simulink model "IEEE30_case"  (R2024b)
settings: Solver=FixedStepAuto  StartTime=0  StopTime=5  FixedStep=1e-7  RelTol=1e-3
values from neighbouring files (symbols this model uses):
  GFL_DFIG_7_C_bus = 0.08    [IEEE30_case_parameters.m]
  GFL_DFIG_7_D_mutual = 2.500000e+3    (= 2500)    [IEEE30_case_parameters.m]
  GFL_DFIG_7_f0 = 60    [IEEE30_case_parameters.m]
  GFL_DFIG_7_gPLLi = 3200    [IEEE30_case_parameters.m]
  GFL_DFIG_7_gPLLp = 650    [IEEE30_case_parameters.m]
  GFL_DFIG_7_H_WT = 0.4    [IEEE30_case_parameters.m]
  GFL_DFIG_7_Hg = 0.8    [IEEE30_case_parameters.m]
  GFL_DFIG_7_Igq_ref = 0    [IEEE30_case_parameters.m]
  GFL_DFIG_7_Ird_ref = 704.45696    [IEEE30_case_parameters.m]
  GFL_DFIG_7_KI_V = -300000    [IEEE30_case_parameters.m]
  GFL_DFIG_7_KP_V = -1000    [IEEE30_case_parameters.m]
  GFL_DFIG_7_Ksh = 1.254300e+4    (= 12543)    [IEEE30_case_parameters.m]
  GFL_DFIG_7_Lg = 0.000483    [IEEE30_case_parameters.m]
  GFL_DFIG_7_Lm_pu = 4    [IEEE30_case_parameters.m]
  GFL_DFIG_7_N = 100    [IEEE30_case_parameters.m]
  GFL_DFIG_7_p = 2    [IEEE30_case_parameters.m]
  GFL_DFIG_7_Pitch = 0    [IEEE30_case_parameters.m]
  GFL_DFIG_7_R = 44    [IEEE30_case_parameters.m]
  GFL_DFIG_7_Rg = 2.000000e-5    (= 2e-05)    [IEEE30_case_parameters.m]
  GFL_DFIG_7_rho = 1.225    [IEEE30_case_parameters.m]
  GFL_DFIG_7_rPLLi = 4500    [IEEE30_case_parameters.m]
  GFL_DFIG_7_rPLLp = 620    [IEEE30_case_parameters.m]
  GFL_DFIG_7_Rs_pu = 0.011    [IEEE30_case_parameters.m]
  GFL_DFIG_7_Sbase = 2.000000e+6    (= 2000000)    [IEEE30_case_parameters.m]
  GFL_DFIG_7_ugq_ref = 0    [IEEE30_case_parameters.m]
  GFL_DFIG_7_usd_ref = 0    [IEEE30_case_parameters.m]
  GFL_DFIG_7_Vbase = 690    [IEEE30_case_parameters.m]
  GFL_DFIG_7_Vdc_ref = 1200    [IEEE30_case_parameters.m]
  GFL_DFIG_7_wind = 12    [IEEE30_case_parameters.m]
  GFL_DFIG_7_wm_ref = 518.184209    [IEEE30_case_parameters.m]
  SG_D_13_D = 0.01056    [IEEE30_case_parameters.m]
  SG_D_13_EnableSaturation = 0    [IEEE30_case_parameters.m]
  SG_D_13_f0 = 60    [IEEE30_case_parameters.m]
  SG_D_13_H = 7.5    [IEEE30_case_parameters.m]
  SG_D_13_K_A = 20    [IEEE30_case_parameters.m]
  SG_D_13_K_E = 1.000000e+1    (= 10)    [IEEE30_case_parameters.m]
  SG_D_13_K_F = 2.363    [IEEE30_case_parameters.m]
  SG_D_13_K_s = 0.5    [IEEE30_case_parameters.m]
  SG_D_13_R_a = 0.001088    [IEEE30_case_parameters.m]
  SG_D_13_S_A = 1    [IEEE30_case_parameters.m]
  SG_D_13_S_B = 0.103    [IEEE30_case_parameters.m]
  SG_D_13_S_N = 10.659857    [IEEE30_case_parameters.m]
  SG_D_13_SpeedPara = 200    [IEEE30_case_parameters.m]
  SG_D_13_T_0 = 0.370163    [IEEE30_case_parameters.m]
  SG_D_13_T_1 = 0.3    [IEEE30_case_parameters.m]
  SG_D_13_T_2 = 0.05    [IEEE30_case_parameters.m]
  SG_D_13_T_3 = 0.02    [IEEE30_case_parameters.m]
  SG_D_13_T_4 = 0.005    [IEEE30_case_parameters.m]
  SG_D_13_T_A = 0.02    [IEEE30_case_parameters.m]
  SG_D_13_T_dd = 8.000000e+0    (= 8)    [IEEE30_case_parameters.m]
  SG_D_13_T_ddd = 0.04    [IEEE30_case_parameters.m]
  SG_D_13_T_E = 0.314    [IEEE30_case_parameters.m]
  SG_D_13_T_F = 0.35    [IEEE30_case_parameters.m]
  SG_D_13_T_qd = 0.8    [IEEE30_case_parameters.m]
  SG_D_13_T_qdd = 0.02    [IEEE30_case_parameters.m]
  SG_D_13_T_speed = 0.1    [IEEE30_case_parameters.m]
  SG_D_13_T_w = 0.5    [IEEE30_case_parameters.m]
  SG_D_13_V_ref = 1.696619    [IEEE30_case_parameters.m]
  SG_D_13_w_ref = 376.991118    [IEEE30_case_parameters.m]
  SG_D_13_x_d = 1.9    [IEEE30_case_parameters.m]
  SG_D_13_x_dd = 0.302    [IEEE30_case_parameters.m]
  SG_D_13_x_ddd = 0.204    [IEEE30_case_parameters.m]
  SG_D_13_x_l = 0.05    [IEEE30_case_parameters.m]
  SG_D_13_x_q = 1.3    [IEEE30_case_parameters.m]
  SG_D_13_x_qd = 0.5    [IEEE30_case_parameters.m]
  SG_D_13_x_qdd = 0.3    [IEEE30_case_parameters.m]
  SG_D_1_D = 0.01056    [IEEE30_case_parameters.m]
  SG_D_1_EnableSaturation = 0    [IEEE30_case_parameters.m]
  SG_D_1_f0 = 60    [IEEE30_case_parameters.m]
  SG_D_1_H = 7.5    [IEEE30_case_parameters.m]
  SG_D_1_K_A = 20    [IEEE30_case_parameters.m]
  SG_D_1_K_E = 1.000000e+1    (= 10)    [IEEE30_case_parameters.m]
  SG_D_1_K_F = 2.363    [IEEE30_case_parameters.m]
  SG_D_1_K_s = 0.5    [IEEE30_case_parameters.m]
  SG_D_1_R_a = 0.001088    [IEEE30_case_parameters.m]
  SG_D_1_S_A = 1    [IEEE30_case_parameters.m]
  SG_D_1_S_B = 0.103    [IEEE30_case_parameters.m]
  SG_D_1_S_N = 10.659857    [IEEE30_case_parameters.m]
  SG_D_1_SpeedPara = 200    [IEEE30_case_parameters.m]
  SG_D_1_T_0 = 0.259812    [IEEE30_case_parameters.m]
  SG_D_1_T_1 = 0.3    [IEEE30_case_parameters.m]
  SG_D_1_T_2 = 0.05    [IEEE30_case_parameters.m]
  SG_D_1_T_3 = 0.02    [IEEE30_case_parameters.m]
  SG_D_1_T_4 = 0.005    [IEEE30_case_parameters.m]
  SG_D_1_T_A = 0.02    [IEEE30_case_parameters.m]
  SG_D_1_T_dd = 8.000000e+0    (= 8)    [IEEE30_case_parameters.m]
  SG_D_1_T_ddd = 0.04    [IEEE30_case_parameters.m]
  SG_D_1_T_E = 0.314    [IEEE30_case_parameters.m]
  SG_D_1_T_F = 0.35    [IEEE30_case_parameters.m]
  SG_D_1_T_qd = 0.8    [IEEE30_case_parameters.m]
  SG_D_1_T_qdd = 0.02    [IEEE30_case_parameters.m]
  SG_D_1_T_speed = 0.1    [IEEE30_case_parameters.m]
  SG_D_1_T_w = 0.5    [IEEE30_case_parameters.m]
  SG_D_1_V_ref = 1.544107    [IEEE30_case_parameters.m]
  SG_D_1_w_ref = 376.991118    [IEEE30_case_parameters.m]
  SG_D_1_x_d = 1.9    [IEEE30_case_parameters.m]
  SG_D_1_x_dd = 0.302    [IEEE30_case_parameters.m]
  SG_D_1_x_ddd = 0.204    [IEEE30_case_parameters.m]
  SG_D_1_x_l = 0.05    [IEEE30_case_parameters.m]
  SG_D_1_x_q = 1.3    [IEEE30_case_parameters.m]
  SG_D_1_x_qd = 0.5    [IEEE30_case_parameters.m]
  SG_D_1_x_qdd = 0.3    [IEEE30_case_parameters.m]
  SG_D_22_D = 0.01056    [IEEE30_case_parameters.m]
  SG_D_22_EnableSaturation = 0    [IEEE30_case_parameters.m]
  SG_D_22_f0 = 60    [IEEE30_case_parameters.m]
  SG_D_22_H = 7.5    [IEEE30_case_parameters.m]
  SG_D_22_K_A = 20    [IEEE30_case_parameters.m]
  SG_D_22_K_E = 1.000000e+1    (= 10)    [IEEE30_case_parameters.m]
  SG_D_22_K_F = 2.363    [IEEE30_case_parameters.m]
  SG_D_22_K_s = 0.5    [IEEE30_case_parameters.m]
  SG_D_22_R_a = 0.001088    [IEEE30_case_parameters.m]
  SG_D_22_S_A = 1    [IEEE30_case_parameters.m]
  SG_D_22_S_B = 0.103    [IEEE30_case_parameters.m]
  SG_D_22_S_N = 10.659857    [IEEE30_case_parameters.m]
  SG_D_22_SpeedPara = 200    [IEEE30_case_parameters.m]
  SG_D_22_T_0 = 0.216121    [IEEE30_case_parameters.m]
  SG_D_22_T_1 = 0.3    [IEEE30_case_parameters.m]
  SG_D_22_T_2 = 0.05    [IEEE30_case_parameters.m]
  SG_D_22_T_3 = 0.02    [IEEE30_case_parameters.m]
  SG_D_22_T_4 = 0.005    [IEEE30_case_parameters.m]
  ... (+126 more)
(part 17 of 27)

== system IEEE30_case/SG_D_1/d_psi_kq_SG_D_1_block ==
  note: d_psi_kq_SG_D_1 in IEEE30_case
      | $-\frac{\psi _{\mathrm{gq},\mathrm{SG},D,1}+\psi _{\mathrm{kq},\mathrm{SG},D,1}+\frac{\left(x_{l}-x_{\mathrm{qd}}\right)\,\left(\psi _{q,\mathrm{SG},D,1}+\frac{\psi _{\mathrm{gq},\mathrm{SG},D,1}\,\left(x_{l}-x_{\mathrm{qdd}}\right)}{x_{l}-x_{\mathrm{qd}}}+\frac{\psi _{\mathrm{kq},\mathrm{SG},D,1}\,\left(x_{\mathrm{qd}}-x_{\mathrm{qdd}}\right)}{x_{l}-x_{\mathrm{qd}}}\right)}{x_{\mathrm{qdd}}}}{T_{\mathrm{qdd}}}$
      | Automatically generated on 2025-11-01 18:30:18 .
  State_psi_gq_SG_D_1_66a42 : Inport
  State_psi_kq_SG_D_1_f6edb : Inport  Port=2
  State_psi_gq_SG_D_1_3bf06 : Inport  Port=3
  State_psi_kq_SG_D_1_b2a24 : Inport  Port=4
  State_psi_q_SG_D_1_f72b4 : Inport  Port=5
  Add_37b64 : Sum
  Add_70e19 : Sum
  Add_86bb6 : Sum
  Add_caec9 : Sum
  Add_e8957 : Sum
  Add_f96b5 : Sum
  Constant_-1_1ee71 : Constant  Value=-1
  Constant_-1_42dcf : Constant  Value=-1
  Constant_-1_ae184 : Constant  Value=-1
  Constant_-1_b39c3 : Constant  Value=-1
  Constant_-1_df8ac : Constant  Value=-1
  Constant_T_qdd_72f05 : Constant  Value=T_qdd
  Constant_x_l_0c777 : Constant  Value=x_l
  Constant_x_l_15b0a : Constant  Value=x_l
  Constant_x_l_3ca11 : Constant  Value=x_l
  Constant_x_l_4ff6a : Constant  Value=x_l
  Constant_x_qd_677f8 : Constant  Value=x_qd
  Constant_x_qd_b6ebb : Constant  Value=x_qd
  Constant_x_qd_d4607 : Constant  Value=x_qd
  Constant_x_qd_dcc1d : Constant  Value=x_qd
  Constant_x_qdd_61ea3 : Constant  Value=x_qdd
  Constant_x_qdd_8287c : Constant  Value=x_qdd
  Constant_x_qdd_95e13 : Constant  Value=x_qdd
  Divide_1c15d : Product  Inputs=*/
  Divide_39d85 : Product  Inputs=*/
  Divide_cbd1b : Product  Inputs=*/
  Divide_e3ee2 : Product  Inputs=*/
  Product_05f1c : Product
  Product_6315e : Product
  Product_6a7e9 : Product
  Product_6f561 : Product
  Product_70210 : Product
  Product_d8668 : Product
  Product_e096e : Product
  Product_f70fb : Product
  Subtract_2999a : Sum  Inputs=+-
  Subtract_5330c : Sum  Inputs=+-
  Subtract_efeff : Sum  Inputs=+-
  Blockout_d_psi_kq_SG_D_1_05b7c : Outport
  wires:
  Product_6f561/1 -> Add_caec9/1
  Constant_-1_ae184/1 -> Product_6f561/1
  Constant_x_l_15b0a/1 -> Product_6f561/2
  Constant_x_qdd_95e13/1 -> Add_caec9/2
  Constant_-1_df8ac/1 -> Product_70210/1
  Constant_x_qd_677f8/1 -> Subtract_5330c/1
  Constant_x_qd_d4607/1 -> Add_86bb6/2
  Constant_-1_1ee71/1 -> Product_e096e/1
  Constant_x_l_4ff6a/1 -> Product_70210/2
  Constant_x_qdd_8287c/1 -> Subtract_5330c/2
  Constant_x_qd_b6ebb/1 -> Add_f96b5/2
  Constant_x_l_0c777/1 -> Product_e096e/2
  Subtract_2999a/1 -> Add_37b64/1
  Product_f70fb/1 -> Subtract_2999a/1
  State_psi_gq_SG_D_1_3bf06/1 -> Product_d8668/1
  Add_caec9/1 -> Product_d8668/2
  Product_e096e/1 -> Add_e8957/1
  Constant_x_qd_dcc1d/1 -> Add_e8957/2
  State_psi_kq_SG_D_1_b2a24/1 -> Product_05f1c/1
  Product_70210/1 -> Add_f96b5/1
  Subtract_5330c/1 -> Product_05f1c/2
  Product_d8668/1 -> Divide_e3ee2/1
  Add_e8957/1 -> Divide_e3ee2/2
  Product_05f1c/1 -> Divide_39d85/1
  Add_f96b5/1 -> Divide_39d85/2
  Constant_-1_b39c3/1 -> Product_6315e/1
  Constant_x_l_3ca11/1 -> Product_6315e/2
  Divide_e3ee2/1 -> Subtract_efeff/1
  Divide_39d85/1 -> Subtract_efeff/2
  Product_6315e/1 -> Add_86bb6/1
  Add_70e19/1 -> Product_6a7e9/2
  Subtract_efeff/1 -> Add_70e19/1
  State_psi_q_SG_D_1_f72b4/1 -> Add_70e19/2
  Constant_-1_42dcf/1 -> Product_f70fb/1
  State_psi_gq_SG_D_1_66a42/1 -> Product_f70fb/2
  Divide_1c15d/1 -> Add_37b64/2
  Product_6a7e9/1 -> Divide_1c15d/1
  Add_86bb6/1 -> Product_6a7e9/1
  State_psi_kq_SG_D_1_f6edb/1 -> Subtract_2999a/2
  Constant_x_qdd_61ea3/1 -> Divide_1c15d/2
  Add_37b64/1 -> Divide_cbd1b/1
  Constant_T_qdd_72f05/1 -> Divide_cbd1b/2
  Divide_cbd1b/1 -> Blockout_d_psi_kq_SG_D_1_05b7c/1

== system IEEE30_case/SG_D_1/d_psi_q_SG_D_1_block ==
  note: d_psi_q_SG_D_1 in IEEE30_case
      | $2\,\pi \,f_{0}\,\left(v_{d,\mathrm{SG},D,1}\,\cos\left(\theta _{\mathrm{SG},D,1}\right)+v_{q,\mathrm{SG},D,1}\,\sin\left(\theta _{\mathrm{SG},D,1}\right)-\frac{R_{a}\,\left(\psi _{q,\mathrm{SG},D,1}+\frac{\psi _{\mathrm{gq},\mathrm{SG},D,1}\,\left(x_{l}-x_{\mathrm{qdd}}\right)}{x_{l}-x_{\mathrm{qd}}}+\frac{\psi _{\mathrm{kq},\mathrm{SG},D,1}\,\left(x_{\mathrm{qd}}-x_{\mathrm{qdd}}\right)}{x_{l}-x_{\mathrm{qd}}}\right)}{x_{\mathrm{qdd}}}-\frac{\psi _{d,\mathrm{SG},D,1}\,w_{\mathrm{SG},D,1}}{2\,f_{0}\,\pi }\right)$
      | Automatically generated on 2025-11-01 18:30:00 .
  State_psi_gq_SG_D_1_26e24 : Inport
  State_psi_kq_SG_D_1_f77dd : Inport  Port=2
  State_psi_q_SG_D_1_070ab : Inport  Port=3
  Input_v_d_SG_D_1_1c698 : Inport  Port=4
  State_theta_SG_D_1_9525e : Inport  Port=5
  Input_v_q_SG_D_1_e75ba : Inport  Port=6
  State_theta_SG_D_1_5ff34 : Inport  Port=7
  State_psi_d_SG_D_1_80a58 : Inport  Port=8
  State_w_SG_D_1_948ae : Inport  Port=9
  Add_13797 : Sum
  Add_7e781 : Sum
  Add_babbf : Sum
  Add_e7483 : Sum
  Add_fa18c : Sum
  Constant_-1_3c07d : Constant  Value=-1
  Constant_-1_59b7b : Constant  Value=-1
  Constant_-1_b49b8 : Constant  Value=-1
  Constant_-2.0_d7f57 : Constant  Value=-2.0
  Constant_2.0_efb3f : Constant  Value=2.0
  Constant_R_a_8a746 : Constant  Value=R_a
  Constant_f0_40920 : Constant  Value=f0
  Constant_f0_9936c : Constant  Value=f0
  Constant_pi_9d2f0 : Constant  Value=pi
  Constant_pi_b54fb : Constant  Value=pi
  Constant_x_l_786db : Constant  Value=x_l
  Constant_x_l_8a064 : Constant  Value=x_l
  Constant_x_l_f0cc6 : Constant  Value=x_l
  Constant_x_qd_30d34 : Constant  Value=x_qd
  Constant_x_qd_33bbe : Constant  Value=x_qd
  Constant_x_qd_7c0de : Constant  Value=x_qd
  Constant_x_qdd_2670b : Constant  Value=x_qdd
  Constant_x_qdd_2fe7a : Constant  Value=x_qdd
  Constant_x_qdd_833e6 : Constant  Value=x_qdd
  Divide_25523 : Product  Inputs=*/
  Divide_748df : Product  Inputs=*/
  Divide_82d73 : Product  Inputs=*/
  Divide_b6ace : Product  Inputs=*/
  MathFunc_cos_34627 : Trigonometry  Operator=cos
  MathFunc_sin_db86f : Trigonometry
  Product_09f90 : Product
  Product_7c18a : Product
  Product_813ef : Product
  Product_93581 : Product
  Product_a2672 : Product
  Product_a434f : Product
  Product_c21a3 : Product
  Product_c33c2 : Product
  Product_c7474 : Product
  Product_edeb5 : Product
  Product_f09fe : Product
  Product_f2590 : Product
  Product_f523a : Product
  Product_fbfd0 : Product
  Subtract_2dac9 : Sum  Inputs=+-
  Subtract_4a509 : Sum  Inputs=+-
  Subtract_587b4 : Sum  Inputs=+-
  Subtract_81de1 : Sum  Inputs=+-
  Blockout_d_psi_q_SG_D_1_abfd1 : Outport
  wires:
  Divide_b6ace/1 -> Subtract_587b4/1
  Product_f09fe/1 -> Add_e7483/1
  Constant_x_l_786db/1 -> Product_f09fe/2
  Constant_-1_3c07d/1 -> Product_f09fe/1
  Constant_x_qdd_2fe7a/1 -> Add_e7483/2
  Constant_x_l_f0cc6/1 -> Product_09f90/2
  Constant_-1_b49b8/1 -> Product_09f90/1
  Constant_x_l_8a064/1 -> Product_edeb5/2
  Constant_x_qdd_2670b/1 -> Subtract_81de1/2
  State_psi_kq_SG_D_1_f77dd/1 -> Product_f2590/1
  Constant_-1_59b7b/1 -> Product_edeb5/1
  Constant_x_qd_33bbe/1 -> Subtract_81de1/1
  State_psi_gq_SG_D_1_26e24/1 -> Product_a2672/1
  Product_c7474/1 -> Blockout_d_psi_q_SG_D_1_abfd1/1
  Subtract_587b4/1 -> Add_fa18c/1
  Product_a2672/1 -> Divide_b6ace/1
  Add_e7483/1 -> Product_a2672/2
  Divide_748df/1 -> Subtract_587b4/2
  Product_09f90/1 -> Add_babbf/1
  Constant_x_qd_30d34/1 -> Add_babbf/2
  Constant_-2.0_d7f57/1 -> Product_fbfd0/1
  Product_f2590/1 -> Divide_748df/1
  Product_edeb5/1 -> Add_13797/1
  Subtract_81de1/1 -> Product_f2590/2
  Constant_x_qd_7c0de/1 -> Add_13797/2
  Add_babbf/1 -> Divide_b6ace/2
  Add_13797/1 -> Divide_748df/2
  Constant_f0_40920/1 -> Product_f523a/2
  State_psi_q_SG_D_1_070ab/1 -> Add_fa18c/2
  Product_c21a3/1 -> Product_813ef/1
  Constant_R_a_8a746/1 -> Product_7c18a/1
  Product_813ef/1 -> Divide_82d73/2
  Product_7c18a/1 -> Divide_25523/1
  Add_fa18c/1 -> Product_7c18a/2
  State_theta_SG_D_1_9525e/1 -> MathFunc_cos_34627/1
  Input_v_d_SG_D_1_1c698/1 -> Product_c33c2/1
  Constant_x_qdd_833e6/1 -> Divide_25523/2
  MathFunc_cos_34627/1 -> Product_c33c2/2
  State_theta_SG_D_1_5ff34/1 -> MathFunc_sin_db86f/1
  Divide_25523/1 -> Subtract_2dac9/1
  Constant_2.0_efb3f/1 -> Product_c21a3/1
  State_w_SG_D_1_948ae/1 -> Product_93581/2
  Constant_pi_9d2f0/1 -> Product_c21a3/2
  Subtract_4a509/1 -> Add_7e781/1
  Product_c33c2/1 -> Subtract_2dac9/2
  Divide_82d73/1 -> Add_7e781/2
  Input_v_q_SG_D_1_e75ba/1 -> Product_a434f/1
  MathFunc_sin_db86f/1 -> Product_a434f/2
  Product_a434f/1 -> Subtract_4a509/2
  State_psi_d_SG_D_1_80a58/1 -> Product_93581/1
  Constant_f0_9936c/1 -> Product_813ef/2
  Constant_pi_b54fb/1 -> Product_fbfd0/2
  Subtract_2dac9/1 -> Subtract_4a509/1
  Product_93581/1 -> Divide_82d73/1
  Product_fbfd0/1 -> Product_f523a/1
  Product_f523a/1 -> Product_c7474/1
  Add_7e781/1 -> Product_c7474/2

== system IEEE30_case/SG_D_1/d_theta_SG_D_1_block ==
  note: d_theta_SG_D_1 in IEEE30_case
      | $w_{\mathrm{SG},D,1}-2\,\pi \,f_{0}$
      | Automatically generated on 2025-11-01 18:30:25 .
  State_w_SG_D_1_25fe5 : Inport
  Add_14687 : Sum
  Constant_-2.0_add39 : Constant  Value=-2.0
  Constant_f0_f3afc : Constant  Value=f0
  Constant_pi_ba5a1 : Constant  Value=pi
  Product_57019 : Product
  Product_88f41 : Product
  Blockout_d_theta_SG_D_1_b4601 : Outport
  wires:
  State_w_SG_D_1_25fe5/1 -> Add_14687/2
  Constant_-2.0_add39/1 -> Product_88f41/1
  Constant_f0_f3afc/1 -> Product_57019/2
  Constant_pi_ba5a1/1 -> Product_88f41/2
  Product_57019/1 -> Add_14687/1
  Product_88f41/1 -> Product_57019/1
  Add_14687/1 -> Blockout_d_theta_SG_D_1_b4601/1

== system IEEE30_case/SG_D_1/d_w_SG_D_1_block ==
  note: d_w_SG_D_1 in IEEE30_case
      | $\frac{2\,\pi \,T_{m,\mathrm{SG},D,1}\,f_{0}-D\,\left(w_{\mathrm{SG},D,1}-2\,\pi \,f_{0}\right)+2\,\pi \,f_{0}\,\left(\frac{\psi _{d,\mathrm{SG},D,1}\,\left(\psi _{q,\mathrm{SG},D,1}+\frac{\psi _{\mathrm{gq},\mathrm{SG},D,1}\,\left(x_{l}-x_{\mathrm{qdd}}\right)}{x_{l}-x_{\mathrm{qd}}}+\frac{\psi _{\mathrm{kq},\mathrm{SG},D,1}\,\left(x_{\mathrm{qd}}-x_{\mathrm{qdd}}\right)}{x_{l}-x_{\mathrm{qd}}}\right)}{x_{\mathrm{qdd}}}+\frac{\psi _{q,\mathrm{SG},D,1}\,\left(\frac{\psi _{\mathrm{1d},\mathrm{SG},D,1}\,\left(x_{\mathrm{dd}}-x_{\mathrm{ddd}}\right)}{x_{\mathrm{dd}}-x_{l}}-\psi _{d,\mathrm{SG},D,1}+\frac{\psi _{\mathrm{fd},\mathrm{SG},D,1}\,\left(x_{\mathrm{ddd}}-x_{l}\right)}{x_{\mathrm{dd}}-x_{l}}\right)}{x_{\mathrm{ddd}}}\right)}{2\,H}$
      | Automatically generated on 2025-11-01 18:30:23 .
  State_w_SG_D_1_7370e : Inport
  State_T_m_SG_D_1_0f890 : Inport  Port=2
  State_psi_d_SG_D_1_f033d : Inport  Port=3
  State_psi_gq_SG_D_1_ce49a : Inport  Port=4
  State_psi_kq_SG_D_1_2014b : Inport  Port=5
  State_psi_q_SG_D_1_d909e : Inport  Port=6
  State_psi_q_SG_D_1_91429 : Inport  Port=7
  State_psi_1d_SG_D_1_f2003 : Inport  Port=8
  State_psi_d_SG_D_1_182c7 : Inport  Port=9
  State_psi_fd_SG_D_1_cb4ff : Inport  Port=10
  Add_1b04e : Sum
  Add_3c3c4 : Sum
  Add_504a4 : Sum
  Add_52c35 : Sum
  Add_7a12c : Sum
  Add_93399 : Sum
  Add_cb8c9 : Sum
  Add_f05de : Sum
  Constant_-1_0111a : Constant  Value=-1
  Constant_-1_26c51 : Constant  Value=-1
  Constant_-1_4576b : Constant  Value=-1
  Constant_-1_50060 : Constant  Value=-1
  Constant_-1_ad6c8 : Constant  Value=-1
  Constant_-1_eb116 : Constant  Value=-1
  Constant_-2.0_547f8 : Constant  Value=-2.0
  Constant_2.0_1c04a : Constant  Value=2.0
  Constant_2.0_a4d1c : Constant  Value=2.0
  Constant_2.0_f8b7f : Constant  Value=2.0
  Constant_D_d7036 : Constant  Value=D
  Constant_H_554eb : Constant  Value=H
  Constant_f0_0096c : Constant  Value=f0
  Constant_f0_2940f : Constant  Value=f0
  Constant_f0_69a0e : Constant  Value=f0
  Constant_pi_0f87c : Constant  Value=pi
  Constant_pi_319c6 : Constant  Value=pi
  Constant_pi_8e62b : Constant  Value=pi
  Constant_x_dd_309c9 : Constant  Value=x_dd
  Constant_x_dd_3432c : Constant  Value=x_dd
  Constant_x_dd_facee : Constant  Value=x_dd
  Constant_x_ddd_3db31 : Constant  Value=x_ddd
  Constant_x_ddd_3eae1 : Constant  Value=x_ddd
  Constant_x_ddd_ff935 : Constant  Value=x_ddd
  Constant_x_l_2cb1f : Constant  Value=x_l
  Constant_x_l_84837 : Constant  Value=x_l
  Constant_x_l_9b1db : Constant  Value=x_l
  Constant_x_l_a64bd : Constant  Value=x_l
  Constant_x_l_e4a07 : Constant  Value=x_l
  Constant_x_l_e9bb8 : Constant  Value=x_l
  Constant_x_qd_17ed2 : Constant  Value=x_qd
  Constant_x_qd_23798 : Constant  Value=x_qd
  Constant_x_qd_dc38f : Constant  Value=x_qd
  Constant_x_qdd_2bc67 : Constant  Value=x_qdd
  Constant_x_qdd_78861 : Constant  Value=x_qdd
  Constant_x_qdd_800f4 : Constant  Value=x_qdd
  Divide_127ba : Product  Inputs=*/
  Divide_2cfe5 : Product  Inputs=*/
  Divide_63b05 : Product  Inputs=*/
  Divide_642c5 : Product  Inputs=*/
  Divide_97c4a : Product  Inputs=*/
  Divide_b46f1 : Product  Inputs=*/
  Divide_d4016 : Product  Inputs=*/
  Product_0933f : Product
  Product_0fac4 : Product
  Product_1006a : Product
  Product_1dcb5 : Product
  Product_326c4 : Product
  Product_38155 : Product
  Product_5f295 : Product
  Product_68df4 : Product
  Product_69256 : Product
  Product_7cfa6 : Product
  Product_80476 : Product
  Product_83fd3 : Product
  Product_934cb : Product
  Product_9c84a : Product
  Product_c0ac4 : Product
  Product_c2018 : Product
  Product_c5be4 : Product
  Product_cf201 : Product
  Product_eb15b : Product
  Product_eec16 : Product
  Product_efe5f : Product
  Product_f8974 : Product
  Subtract_025ed : Sum  Inputs=+-
  Subtract_1f74c : Sum  Inputs=+-
  Subtract_60322 : Sum  Inputs=+-
  Subtract_6c086 : Sum  Inputs=+-
  Subtract_9075a : Sum  Inputs=+-
  Subtract_9a40e : Sum  Inputs=+-
  Subtract_abe5e : Sum  Inputs=+-
  Subtract_de9cb : Sum  Inputs=+-
  Blockout_d_w_SG_D_1_18f98 : Outport
  wires:
  Product_0933f/1 -> Add_3c3c4/1
  Constant_-1_0111a/1 -> Product_f8974/1
  Constant_pi_8e62b/1 -> Product_326c4/2
  Constant_x_qdd_2bc67/1 -> Add_f05de/2
  Constant_x_l_e4a07/1 -> Product_f8974/2
  Product_f8974/1 -> Add_f05de/1
  Constant_x_qd_23798/1 -> Subtract_9a40e/1
  Constant_-1_26c51/1 -> Product_5f295/1
  Product_c5be4/1 -> Product_0933f/1
  Constant_x_qdd_800f4/1 -> Subtract_9a40e/2
  State_psi_q_SG_D_1_91429/1 -> Product_38155/1
  Constant_x_l_e9bb8/1 -> Product_5f295/2
  Constant_-1_4576b/1 -> Product_1dcb5/1
  Constant_x_l_84837/1 -> Product_1dcb5/2
  Constant_-1_50060/1 -> Product_cf201/1
  Product_5f295/1 -> Add_93399/1
  State_psi_1d_SG_D_1_f2003/1 -> Product_cf201/2
  Constant_x_dd_3432c/1 -> Subtract_1f74c/1
  Subtract_9a40e/1 -> Product_68df4/2
  Constant_x_ddd_ff935/1 -> Subtract_1f74c/2
  State_psi_gq_SG_D_1_ce49a/1 -> Product_eec16/1
  Product_80476/1 -> Product_efe5f/1
  Add_f05de/1 -> Product_eec16/2
  Constant_x_qd_dc38f/1 -> Add_93399/2
  State_psi_kq_SG_D_1_2014b/1 -> Product_68df4/1
  Constant_f0_2940f/1 -> Product_0933f/2
  Product_1dcb5/1 -> Add_52c35/1
  Constant_x_dd_309c9/1 -> Subtract_025ed/1
  Constant_x_qd_17ed2/1 -> Add_52c35/2
  Product_cf201/1 -> Product_c2018/1
  Subtract_1f74c/1 -> Product_c2018/2
  Constant_x_l_2cb1f/1 -> Subtract_025ed/2
  Constant_x_ddd_3db31/1 -> Subtract_9075a/1
  Constant_x_l_9b1db/1 -> Subtract_9075a/2
  State_w_SG_D_1_7370e/1 -> Add_3c3c4/2
  Divide_642c5/1 -> Add_cb8c9/1
  Constant_-1_ad6c8/1 -> Product_69256/1
  Product_eec16/1 -> Divide_97c4a/1
  Add_3c3c4/1 -> Product_0fac4/2
  Divide_97c4a/1 -> Subtract_60322/1
  Add_93399/1 -> Divide_97c4a/2
  Constant_pi_0f87c/1 -> Product_c5be4/2
  Product_68df4/1 -> Divide_127ba/1
  Add_52c35/1 -> Divide_127ba/2
  Product_c2018/1 -> Divide_2cfe5/1
  Divide_2cfe5/1 -> Add_7a12c/1
  Subtract_025ed/1 -> Divide_2cfe5/2
  State_psi_fd_SG_D_1_cb4ff/1 -> Product_1006a/1
  Subtract_9075a/1 -> Product_1006a/2
  Constant_x_dd_facee/1 -> Subtract_6c086/1
  Constant_x_l_a64bd/1 -> Subtract_6c086/2
  Divide_127ba/1 -> Subtract_60322/2
  Constant_2.0_f8b7f/1 -> Product_326c4/1
  State_psi_d_SG_D_1_182c7/1 -> Add_7a12c/2
  Product_1006a/1 -> Divide_d4016/1
  Subtract_6c086/1 -> Divide_d4016/2
  Constant_-2.0_547f8/1 -> Product_c5be4/1
  Constant_-1_eb116/1 -> Product_80476/1
  State_psi_d_SG_D_1_f033d/1 -> Product_80476/2
  Subtract_60322/1 -> Add_1b04e/1
  Subtract_abe5e/1 -> Product_38155/2
  State_psi_q_SG_D_1_d909e/1 -> Add_1b04e/2
  Add_7a12c/1 -> Subtract_abe5e/1
  Divide_d4016/1 -> Subtract_abe5e/2
  Add_1b04e/1 -> Product_efe5f/2
  Constant_D_d7036/1 -> Product_69256/2
  Product_326c4/1 -> Product_c0ac4/1
  State_T_m_SG_D_1_0f890/1 -> Product_c0ac4/2
  Constant_2.0_1c04a/1 -> Product_eb15b/1
  Constant_pi_319c6/1 -> Product_eb15b/2
  Product_efe5f/1 -> Divide_642c5/1
  Constant_x_qdd_78861/1 -> Divide_642c5/2
  Product_38155/1 -> Divide_b46f1/1
  Constant_x_ddd_3eae1/1 -> Divide_b46f1/2
  Product_69256/1 -> Product_0fac4/1
  Product_c0ac4/1 -> Product_83fd3/1
  Constant_f0_69a0e/1 -> Product_83fd3/2
  Product_eb15b/1 -> Product_934cb/1
  Constant_f0_0096c/1 -> Product_934cb/2
  Divide_b46f1/1 -> Add_cb8c9/2
  Product_0fac4/1 -> Add_504a4/1
  Product_83fd3/1 -> Add_504a4/2
  Product_934cb/1 -> Product_7cfa6/1
  Add_cb8c9/1 -> Product_7cfa6/2
  Add_504a4/1 -> Subtract_de9cb/1
  Product_7cfa6/1 -> Subtract_de9cb/2
  Constant_2.0_a4d1c/1 -> Product_9c84a/1
  Constant_H_554eb/1 -> Product_9c84a/2
  Subtract_de9cb/1 -> Divide_63b05/1
  Product_9c84a/1 -> Divide_63b05/2
  Divide_63b05/1 -> Blockout_d_w_SG_D_1_18f98/1

== system IEEE30_case/SG_D_1/i_d_SG_D_1_block ==
  note: i_d_SG_D_1 in IEEE30_case
      | $\frac{\sin\left(\theta _{\mathrm{SG},D,1}\right)\,\left(\frac{\psi _{\mathrm{1d},\mathrm{SG},D,1}\,\left(x_{\mathrm{dd}}-x_{\mathrm{ddd}}\right)}{x_{\mathrm{dd}}-x_{l}}-\psi _{d,\mathrm{SG},D,1}+\frac{\psi _{\mathrm{fd},\mathrm{SG},D,1}\,\left(x_{\mathrm{ddd}}-x_{l}\right)}{x_{\mathrm{dd}}-x_{l}}\right)}{x_{\mathrm{ddd}}}-\frac{\cos\left(\theta _{\mathrm{SG},D,1}\right)\,\left(\psi _{q,\mathrm{SG},D,1}+\frac{\psi _{\mathrm{gq},\mathrm{SG},D,1}\,\left(x_{l}-x_{\mathrm{qdd}}\right)}{x_{l}-x_{\mathrm{qd}}}+\frac{\psi _{\mathrm{kq},\mathrm{SG},D,1}\,\left(x_{\mathrm{qd}}-x_{\mathrm{qdd}}\right)}{x_{l}-x_{\mathrm{qd}}}\right)}{x_{\mathrm{qdd}}}$
      | Automatically generated on 2025-11-01 18:30:46 .
  State_psi_gq_SG_D_1_10f28 : Inport
  State_psi_kq_SG_D_1_4ef53 : Inport  Port=2
  State_psi_q_SG_D_1_228eb : Inport  Port=3
  State_theta_SG_D_1_e11c7 : Inport  Port=4
  State_psi_1d_SG_D_1_3ebc3 : Inport  Port=5
  State_psi_d_SG_D_1_fb11e : Inport  Port=6
  State_psi_fd_SG_D_1_0507a : Inport  Port=7
  State_theta_SG_D_1_02fe0 : Inport  Port=8
  Add_24308 : Sum
  Add_7a0a2 : Sum
  Add_7a69a : Sum
  Add_d1e5f : Sum
  Add_f0536 : Sum
  Constant_-1_59dde : Constant  Value=-1
  Constant_-1_7abda : Constant  Value=-1
  Constant_-1_a1181 : Constant  Value=-1
  Constant_-1_a17da : Constant  Value=-1
  Constant_-1_b7515 : Constant  Value=-1
  Constant_x_dd_1fa3d : Constant  Value=x_dd
  Constant_x_dd_29f2e : Constant  Value=x_dd
  Constant_x_dd_b64b8 : Constant  Value=x_dd
  Constant_x_ddd_3f9b0 : Constant  Value=x_ddd
  Constant_x_ddd_65959 : Constant  Value=x_ddd
  Constant_x_ddd_c9110 : Constant  Value=x_ddd
  Constant_x_l_9bf54 : Constant  Value=x_l
  Constant_x_l_af929 : Constant  Value=x_l
  Constant_x_l_ba077 : Constant  Value=x_l
  Constant_x_l_d0162 : Constant  Value=x_l
  Constant_x_l_d4392 : Constant  Value=x_l
  Constant_x_l_dba0e : Constant  Value=x_l
  Constant_x_qd_27afc : Constant  Value=x_qd
  Constant_x_qd_954d1 : Constant  Value=x_qd
  Constant_x_qd_e6c88 : Constant  Value=x_qd
  Constant_x_qdd_af3a2 : Constant  Value=x_qdd
  Constant_x_qdd_b8e58 : Constant  Value=x_qdd
  Constant_x_qdd_e9a31 : Constant  Value=x_qdd
  Divide_5a4cd : Product  Inputs=*/
  Divide_67d6f : Product  Inputs=*/
  Divide_a27a7 : Product  Inputs=*/
  Divide_c8470 : Product  Inputs=*/
  Divide_ddfe3 : Product  Inputs=*/
  Divide_f05ae : Product  Inputs=*/
  MathFunc_cos_32500 : Trigonometry  Operator=cos
  MathFunc_sin_c6b27 : Trigonometry
  Product_30c3f : Product
  Product_68f51 : Product
  Product_697c9 : Product
  Product_6b664 : Product
  Product_711f9 : Product
  Product_764be : Product
  Product_81c61 : Product
  Product_abe10 : Product
  Product_c6dcb : Product
  Product_d25e2 : Product
  Product_f59cd : Product
  Subtract_5fee8 : Sum  Inputs=+-
  Subtract_6f256 : Sum  Inputs=+-
  Subtract_853c5 : Sum  Inputs=+-
  Subtract_9c843 : Sum  Inputs=+-
  Subtract_a3c45 : Sum  Inputs=+-
  Subtract_aaa91 : Sum  Inputs=+-
  Subtract_c699c : Sum  Inputs=+-
  Subtract_d2259 : Sum  Inputs=+-
  Blockout_i_d_SG_D_1_f91f6 : Outport
  wires:
  Constant_-1_7abda/1 -> Product_764be/1
  Constant_x_l_ba077/1 -> Product_764be/2
  Constant_x_ddd_3f9b0/1 -> Subtract_aaa91/2
  Product_764be/1 -> Add_24308/1
  Constant_x_qdd_af3a2/1 -> Subtract_c699c/2
  Constant_x_l_9bf54/1 -> Product_711f9/2
  Constant_x_qd_e6c88/1 -> Add_d1e5f/2
  Constant_x_qdd_b8e58/1 -> Add_24308/2
  Constant_x_qd_954d1/1 -> Subtract_c699c/1
  MathFunc_cos_32500/1 -> Product_c6dcb/2
  Constant_-1_a1181/1 -> Product_711f9/1
  Constant_-1_59dde/1 -> Product_68f51/1
  Subtract_d2259/1 -> Blockout_i_d_SG_D_1_f91f6/1
  Constant_x_l_af929/1 -> Product_68f51/2
  Divide_67d6f/1 -> Subtract_a3c45/1
  State_psi_gq_SG_D_1_10f28/1 -> Product_697c9/1
  Subtract_6f256/1 -> Product_d25e2/2
  Add_24308/1 -> Product_697c9/2
  Divide_c8470/1 -> Add_7a0a2/1
  Product_711f9/1 -> Add_f0536/1
  Constant_x_qd_27afc/1 -> Add_f0536/2
  State_psi_kq_SG_D_1_4ef53/1 -> Product_f59cd/1
  Add_7a0a2/1 -> Subtract_9c843/1
  Add_f0536/1 -> Divide_67d6f/2
  Subtract_c699c/1 -> Product_f59cd/2
  Product_68f51/1 -> Add_d1e5f/1
  Constant_-1_b7515/1 -> Product_30c3f/1
  State_psi_1d_SG_D_1_3ebc3/1 -> Product_30c3f/2
  Constant_x_dd_29f2e/1 -> Subtract_aaa91/1
  Product_697c9/1 -> Divide_67d6f/1
  Product_81c61/1 -> Divide_5a4cd/1
  Subtract_aaa91/1 -> Product_6b664/2
  Product_f59cd/1 -> Divide_ddfe3/1
  Product_30c3f/1 -> Product_6b664/1
  Add_d1e5f/1 -> Divide_ddfe3/2
  Constant_x_dd_1fa3d/1 -> Subtract_853c5/1
  Subtract_a3c45/1 -> Add_7a69a/1
  Constant_x_l_d0162/1 -> Subtract_853c5/2
  Constant_x_ddd_65959/1 -> Subtract_6f256/1
  Constant_x_l_d4392/1 -> Subtract_6f256/2
  Divide_5a4cd/1 -> Subtract_d2259/2
  Divide_ddfe3/1 -> Subtract_a3c45/2
  State_theta_SG_D_1_e11c7/1 -> MathFunc_cos_32500/1
  Product_6b664/1 -> Divide_c8470/1
  Subtract_853c5/1 -> Divide_c8470/2
  State_theta_SG_D_1_02fe0/1 -> MathFunc_sin_c6b27/1
  State_psi_fd_SG_D_1_0507a/1 -> Product_d25e2/1
  Constant_x_dd_b64b8/1 -> Subtract_5fee8/1
  Constant_x_l_dba0e/1 -> Subtract_5fee8/2
  State_psi_q_SG_D_1_228eb/1 -> Add_7a69a/2
  State_psi_d_SG_D_1_fb11e/1 -> Add_7a0a2/2
  Constant_x_ddd_c9110/1 -> Divide_5a4cd/2
  MathFunc_sin_c6b27/1 -> Product_81c61/2
  Product_d25e2/1 -> Divide_f05ae/1
  Constant_-1_a17da/1 -> Product_abe10/1
  Subtract_5fee8/1 -> Divide_f05ae/2
  Add_7a69a/1 -> Product_abe10/2
  Divide_f05ae/1 -> Subtract_9c843/2
  Product_abe10/1 -> Product_c6dcb/1
  Subtract_9c843/1 -> Product_81c61/1
  Constant_x_qdd_e9a31/1 -> Divide_a27a7/2
  Product_c6dcb/1 -> Divide_a27a7/1
  Divide_a27a7/1 -> Subtract_d2259/1

== system IEEE30_case/SG_D_1/i_q_SG_D_1_block ==
  note: i_q_SG_D_1 in IEEE30_case
      | $-\frac{\sin\left(\theta _{\mathrm{SG},D,1}\right)\,\left(\psi _{q,\mathrm{SG},D,1}+\frac{\psi _{\mathrm{gq},\mathrm{SG},D,1}\,\left(x_{l}-x_{\mathrm{qdd}}\right)}{x_{l}-x_{\mathrm{qd}}}+\frac{\psi _{\mathrm{kq},\mathrm{SG},D,1}\,\left(x_{\mathrm{qd}}-x_{\mathrm{qdd}}\right)}{x_{l}-x_{\mathrm{qd}}}\right)}{x_{\mathrm{qdd}}}-\frac{\cos\left(\theta _{\mathrm{SG},D,1}\right)\,\left(\frac{\psi _{\mathrm{1d},\mathrm{SG},D,1}\,\left(x_{\mathrm{dd}}-x_{\mathrm{ddd}}\right)}{x_{\mathrm{dd}}-x_{l}}-\psi _{d,\mathrm{SG},D,1}+\frac{\psi _{\mathrm{fd},\mathrm{SG},D,1}\,\left(x_{\mathrm{ddd}}-x_{l}\right)}{x_{\mathrm{dd}}-x_{l}}\right)}{x_{\mathrm{ddd}}}$
      | Automatically generated on 2025-11-01 18:30:50 .
  State_psi_gq_SG_D_1_d4375 : Inport
  State_psi_kq_SG_D_1_e6fa4 : Inport  Port=2
  State_psi_q_SG_D_1_6d2ce : Inport  Port=3
  State_theta_SG_D_1_9797a : Inport  Port=4
  State_psi_1d_SG_D_1_a42f8 : Inport  Port=5
  State_psi_d_SG_D_1_00c64 : Inport  Port=6
  State_psi_fd_SG_D_1_d5158 : Inport  Port=7
  State_theta_SG_D_1_8458a : Inport  Port=8
  Add_0a10f : Sum
  Add_57d59 : Sum
  Add_a19ba : Sum
  Add_c0cf7 : Sum
  Add_de402 : Sum
  Add_fd0d3 : Sum
  Constant_-1_26e32 : Constant  Value=-1
  Constant_-1_31f17 : Constant  Value=-1
  Constant_-1_52785 : Constant  Value=-1
  Constant_-1_84e32 : Constant  Value=-1
  Constant_-1_b730f : Constant  Value=-1
  Constant_x_dd_04c9e : Constant  Value=x_dd
  Constant_x_dd_8af12 : Constant  Value=x_dd
  Constant_x_dd_8c457 : Constant  Value=x_dd
  Constant_x_ddd_09faa : Constant  Value=x_ddd
  Constant_x_ddd_7b503 : Constant  Value=x_ddd
  Constant_x_ddd_fdb09 : Constant  Value=x_ddd
  Constant_x_l_87bcc : Constant  Value=x_l
  Constant_x_l_91eb9 : Constant  Value=x_l
  Constant_x_l_a2636 : Constant  Value=x_l
  Constant_x_l_afce0 : Constant  Value=x_l
  Constant_x_l_d198f : Constant  Value=x_l
  Constant_x_l_d93d3 : Constant  Value=x_l
  Constant_x_qd_2cc0c : Constant  Value=x_qd
  Constant_x_qd_bf430 : Constant  Value=x_qd
  Constant_x_qd_effc4 : Constant  Value=x_qd
  Constant_x_qdd_9d4e2 : Constant  Value=x_qdd
  Constant_x_qdd_c409e : Constant  Value=x_qdd
  Constant_x_qdd_f5ec5 : Constant  Value=x_qdd
  Divide_04f3a : Product  Inputs=*/
  Divide_14c4e : Product  Inputs=*/
  Divide_16995 : Product  Inputs=*/
  Divide_6bd67 : Product  Inputs=*/
  Divide_77a78 : Product  Inputs=*/
  Divide_eaf94 : Product  Inputs=*/
  MathFunc_cos_65e1a : Trigonometry  Operator=cos
  MathFunc_sin_f9be9 : Trigonometry
  Product_5a536 : Product
  Product_86961 : Product
  Product_901f6 : Product
  Product_95db3 : Product
  Product_9606e : Product
  Product_9d93d : Product
  Product_9e20f : Product
  Product_ac8e4 : Product
  Product_c7d36 : Product
  Product_e9585 : Product
  Product_eb26a : Product
  Subtract_09ffb : Sum  Inputs=+-
  Subtract_16964 : Sum  Inputs=+-
  Subtract_1bfac : Sum  Inputs=+-
  Subtract_36622 : Sum  Inputs=+-
  Subtract_4d30e : Sum  Inputs=+-
  Subtract_e883d : Sum  Inputs=+-
  Subtract_ffe62 : Sum  Inputs=+-
  Blockout_i_q_SG_D_1_159c7 : Outport
  wires:
  State_theta_SG_D_1_8458a/1 -> MathFunc_cos_65e1a/1
  State_psi_fd_SG_D_1_d5158/1 -> Product_5a536/1
  Constant_-1_31f17/1 -> Product_901f6/1
  Constant_x_l_91eb9/1 -> Product_901f6/2
  Subtract_ffe62/1 -> Product_5a536/2
  Constant_x_l_afce0/1 -> Subtract_16964/2
  Product_901f6/1 -> Add_57d59/1
  Constant_x_qdd_9d4e2/1 -> Add_57d59/2
  Constant_x_qd_2cc0c/1 -> Subtract_e883d/1
  Constant_x_qdd_c409e/1 -> Divide_77a78/2
  MathFunc_sin_f9be9/1 -> Product_9d93d/2
  Constant_-1_b730f/1 -> Product_9606e/1
  Constant_x_qdd_f5ec5/1 -> Subtract_e883d/2
  Add_c0cf7/1 -> Product_95db3/2
  Product_ac8e4/1 -> Divide_04f3a/1
  Constant_x_l_a2636/1 -> Product_9606e/2
  Constant_-1_52785/1 -> Product_e9585/1
  Constant_x_l_d198f/1 -> Product_e9585/2
  State_psi_gq_SG_D_1_d4375/1 -> Product_ac8e4/1
  Add_57d59/1 -> Product_ac8e4/2
  Divide_16995/1 -> Add_de402/1
  Product_9606e/1 -> Add_fd0d3/1
  Divide_77a78/1 -> Add_0a10f/1
  Constant_x_qd_effc4/1 -> Add_fd0d3/2
  State_psi_kq_SG_D_1_e6fa4/1 -> Product_9e20f/1
  Add_de402/1 -> Subtract_1bfac/1
  Subtract_e883d/1 -> Product_9e20f/2
  Divide_04f3a/1 -> Subtract_36622/1
  Add_fd0d3/1 -> Divide_04f3a/2
  Product_e9585/1 -> Add_a19ba/1
  Constant_x_qd_bf430/1 -> Add_a19ba/2
  Constant_-1_26e32/1 -> Product_86961/1
  MathFunc_cos_65e1a/1 -> Product_eb26a/2
  Product_5a536/1 -> Divide_eaf94/1
  State_psi_1d_SG_D_1_a42f8/1 -> Product_86961/2
  Constant_x_l_d93d3/1 -> Subtract_09ffb/2
  Constant_x_dd_8af12/1 -> Subtract_4d30e/1
  Divide_eaf94/1 -> Subtract_1bfac/2
  Constant_x_ddd_7b503/1 -> Subtract_4d30e/2
  Product_eb26a/1 -> Divide_6bd67/1
  Product_9e20f/1 -> Divide_14c4e/1
  Product_86961/1 -> Product_c7d36/1
  Add_a19ba/1 -> Divide_14c4e/2
  Subtract_4d30e/1 -> Product_c7d36/2
  State_psi_d_SG_D_1_00c64/1 -> Add_de402/2
  Constant_x_dd_8c457/1 -> Subtract_16964/1
  Constant_x_ddd_09faa/1 -> Subtract_ffe62/1
  Constant_x_l_87bcc/1 -> Subtract_ffe62/2
  Divide_6bd67/1 -> Add_0a10f/2
  Divide_14c4e/1 -> Subtract_36622/2
  State_theta_SG_D_1_9797a/1 -> MathFunc_sin_f9be9/1
  Product_c7d36/1 -> Divide_16995/1
  Subtract_16964/1 -> Divide_16995/2
  Constant_x_dd_04c9e/1 -> Subtract_09ffb/1
  Subtract_36622/1 -> Add_c0cf7/1
  State_psi_q_SG_D_1_6d2ce/1 -> Add_c0cf7/2
  Subtract_09ffb/1 -> Divide_eaf94/2
  Subtract_1bfac/1 -> Product_eb26a/1
  Constant_-1_84e32/1 -> Product_95db3/1
  Product_95db3/1 -> Product_9d93d/1
  Product_9d93d/1 -> Divide_77a78/1
  Constant_x_ddd_fdb09/1 -> Divide_6bd67/2
  Add_0a10f/1 -> Blockout_i_q_SG_D_1_159c7/1

== system IEEE30_case/SG_D_1/theta_SG_D_1_out_block ==
  note: theta_SG_D_1_out in IEEE30_case
      | $\theta _{\mathrm{SG},D,1}$
      | Automatically generated on 2025-11-01 18:30:55 .
  State_theta_SG_D_1_a2930 : Inport
  Blockout_theta_SG_D_1_out_f6ef7 : Outport
  wires:
  State_theta_SG_D_1_a2930/1 -> Blockout_theta_SG_D_1_out_f6ef7/1

== system IEEE30_case/SG_D_1/w_SG_D_1_out_block ==
  note: w_SG_D_1_out in IEEE30_case
      | $w_{\mathrm{SG},D,1}$
      | Automatically generated on 2025-11-01 18:30:55 .
  State_w_SG_D_1_f54e8 : Inport
  Blockout_w_SG_D_1_out_e1973 : Outport
  wires:
  State_w_SG_D_1_f54e8/1 -> Blockout_w_SG_D_1_out_e1973/1

== system IEEE30_case/SG_D_13/T_e_SG_D_13_block ==
  note: T_e_SG_D_13 in IEEE30_case
      | $-\frac{\psi _{d,\mathrm{SG},D,13}\,\left(\psi _{q,\mathrm{SG},D,13}+\frac{\psi _{\mathrm{gq},\mathrm{SG},D,13}\,\left(x_{l}-x_{\mathrm{qdd}}\right)}{x_{l}-x_{\mathrm{qd}}}+\frac{\psi _{\mathrm{kq},\mathrm{SG},D,13}\,\left(x_{\mathrm{qd}}-x_{\mathrm{qdd}}\right)}{x_{l}-x_{\mathrm{qd}}}\right)}{x_{\mathrm{qdd}}}-\frac{\psi _{q,\mathrm{SG},D,13}\,\left(\frac{\psi _{\mathrm{1d},\mathrm{SG},D,13}\,\left(x_{\mathrm{dd}}-x_{\mathrm{ddd}}\right)}{x_{\mathrm{dd}}-x_{l}}-\psi _{d,\mathrm{SG},D,13}+\frac{\psi _{\mathrm{fd},\mathrm{SG},D,13}\,\left(x_{\mathrm{ddd}}-x_{l}\right)}{x_{\mathrm{dd}}-x_{l}}\right)}{x_{\mathrm{ddd}}}$
      | Automatically generated on 2025-11-01 18:35:37 .
  State_psi_d_SG_D_13_06e9a : Inport
  State_psi_gq_SG_D_13_e02fa : Inport  Port=2
  State_psi_kq_SG_D_13_3f4a0 : Inport  Port=3
  State_psi_q_SG_D_13_bdd94 : Inport  Port=4
  State_psi_q_SG_D_13_99ec5 : Inport  Port=5
  State_psi_1d_SG_D_13_43b2f : Inport  Port=6
  State_psi_d_SG_D_13_1b221 : Inport  Port=7
  State_psi_fd_SG_D_13_b4f3b : Inport  Port=8
  Add_02ea9 : Sum
  Add_0e330 : Sum
  Add_7b9af : Sum
  Add_ca388 : Sum
  Add_cda92 : Sum
  Add_d3568 : Sum
  Constant_-1_095fd : Constant  Value=-1
  Constant_-1_32dd9 : Constant  Value=-1
  Constant_-1_5d864 : Constant  Value=-1
  Constant_-1_8577f : Constant  Value=-1
  Constant_-1_c9a45 : Constant  Value=-1
  Constant_x_dd_97ee7 : Constant  Value=x_dd
  Constant_x_dd_a85fb : Constant  Value=x_dd
  Constant_x_dd_db43f : Constant  Value=x_dd
  Constant_x_ddd_57f93 : Constant  Value=x_ddd
  Constant_x_ddd_b5503 : Constant  Value=x_ddd
  Constant_x_ddd_baeed : Constant  Value=x_ddd
  Constant_x_l_1e990 : Constant  Value=x_l
  Constant_x_l_775fb : Constant  Value=x_l
  Constant_x_l_98872 : Constant  Value=x_l
  Constant_x_l_b6163 : Constant  Value=x_l
  Constant_x_l_e4bd4 : Constant  Value=x_l
  Constant_x_l_e6dce : Constant  Value=x_l
  Constant_x_qd_07fae : Constant  Value=x_qd
  Constant_x_qd_54c3d : Constant  Value=x_qd
  Constant_x_qd_fd63a : Constant  Value=x_qd
  Constant_x_qdd_13590 : Constant  Value=x_qdd
  Constant_x_qdd_2c272 : Constant  Value=x_qdd
  Constant_x_qdd_57c10 : Constant  Value=x_qdd
  Divide_029d4 : Product  Inputs=*/
  Divide_11fda : Product  Inputs=*/
  Divide_26293 : Product  Inputs=*/
  Divide_56715 : Product  Inputs=*/
  Divide_8c0fa : Product  Inputs=*/
  Divide_f44ef : Product  Inputs=*/
  Product_0c832 : Product
  Product_16427 : Product
  Product_1fd9e : Product
  Product_33b37 : Product
  Product_366f8 : Product
  Product_3abea : Product
  Product_6086e : Product
  Product_84e6f : Product
  Product_b90aa : Product
  Product_ce8b9 : Product
  Product_f952e : Product
  Subtract_13cd2 : Sum  Inputs=+-
  Subtract_2df29 : Sum  Inputs=+-
  Subtract_66f6c : Sum  Inputs=+-
  Subtract_749d7 : Sum  Inputs=+-
  Subtract_785a3 : Sum  Inputs=+-
  Subtract_ba32e : Sum  Inputs=+-
  Subtract_bb573 : Sum  Inputs=+-
  Blockout_T_e_SG_D_13_a0e2b : Outport
  wires:
  Constant_-1_5d864/1 -> Product_84e6f/1
  Constant_x_l_b6163/1 -> Product_84e6f/2
  Constant_x_l_e4bd4/1 -> Subtract_785a3/2
  Product_84e6f/1 -> Add_0e330/1
  Constant_x_qdd_13590/1 -> Subtract_749d7/2
  Product_ce8b9/1 -> Divide_8c0fa/1
  Constant_x_l_1e990/1 -> Subtract_66f6c/2
  Constant_x_qdd_57c10/1 -> Add_0e330/2
  Product_16427/1 -> Add_d3568/1
  Constant_-1_095fd/1 -> Product_16427/1
  Constant_x_l_98872/1 -> Product_16427/2
  Subtract_749d7/1 -> Product_0c832/2
  Constant_x_ddd_baeed/1 -> Subtract_ba32e/2
  Constant_x_qd_07fae/1 -> Subtract_749d7/1
  Product_33b37/1 -> Add_02ea9/1
  Constant_-1_c9a45/1 -> Product_33b37/1
  Divide_029d4/1 -> Add_ca388/1
  Constant_x_l_e6dce/1 -> Product_33b37/2
  Constant_-1_32dd9/1 -> Product_b90aa/1
  State_psi_1d_SG_D_13_43b2f/1 -> Product_b90aa/2
  Constant_x_dd_a85fb/1 -> Subtract_ba32e/1
  Subtract_2df29/1 -> Product_ce8b9/2
  State_psi_gq_SG_D_13_e02fa/1 -> Product_366f8/1
  Add_0e330/1 -> Product_366f8/2
  Constant_x_qd_fd63a/1 -> Add_d3568/2
  Product_0c832/1 -> Divide_11fda/1
  Product_366f8/1 -> Divide_f44ef/1
  State_psi_kq_SG_D_13_3f4a0/1 -> Product_0c832/1
  Product_1fd9e/1 -> Divide_029d4/1
  Constant_x_qd_54c3d/1 -> Add_02ea9/2
  Product_b90aa/1 -> Product_1fd9e/1
  Constant_-1_8577f/1 -> Product_6086e/1
  Subtract_ba32e/1 -> Product_1fd9e/2
  Constant_x_dd_97ee7/1 -> Subtract_66f6c/1
  Subtract_785a3/1 -> Product_3abea/2
  Constant_x_ddd_b5503/1 -> Subtract_785a3/1
  Add_d3568/1 -> Divide_f44ef/2
  Add_02ea9/1 -> Divide_11fda/2
  Subtract_66f6c/1 -> Divide_029d4/2
  State_psi_q_SG_D_13_bdd94/1 -> Add_7b9af/2
  Product_3abea/1 -> Divide_56715/1
  State_psi_fd_SG_D_13_b4f3b/1 -> Product_3abea/1
  Subtract_bb573/1 -> Divide_56715/2
  Constant_x_dd_db43f/1 -> Subtract_bb573/1
  Constant_x_l_775fb/1 -> Subtract_bb573/2
  Divide_f44ef/1 -> Subtract_13cd2/1
  Divide_11fda/1 -> Subtract_13cd2/2
  State_psi_q_SG_D_13_99ec5/1 -> Product_ce8b9/1
  State_psi_d_SG_D_13_1b221/1 -> Add_ca388/2
  Product_6086e/1 -> Product_f952e/1
  State_psi_d_SG_D_13_06e9a/1 -> Product_6086e/2
  Subtract_13cd2/1 -> Add_7b9af/1
  Add_ca388/1 -> Subtract_2df29/1
  Divide_26293/1 -> Add_cda92/1
  Product_f952e/1 -> Divide_26293/1
  Divide_56715/1 -> Subtract_2df29/2
  Add_7b9af/1 -> Product_f952e/2
  Constant_x_qdd_2c272/1 -> Divide_26293/2
  Constant_x_ddd_57f93/1 -> Divide_8c0fa/2
  Divide_8c0fa/1 -> Add_cda92/2
  Add_cda92/1 -> Blockout_T_e_SG_D_13_a0e2b/1

== system IEEE30_case/SG_D_13/d_E_fd_SG_D_13_block ==
  note: d_E_fd_SG_D_13 in IEEE30_case
      | $\frac{V_{f,\mathrm{SG},D,13}-E_{\mathrm{fd},\mathrm{SG},D,13}\,K_{E}}{T_{E}}$
      | Automatically generated on 2025-11-01 18:35:20 .
  State_E_fd_SG_D_13_5a679 : Inport
  State_V_f_SG_D_13_6d482 : Inport  Port=2
  Add_3e7a5 : Sum
  Constant_-1_49c12 : Constant  Value=-1
  Constant_K_E_3df9a : Constant  Value=K_E
  Constant_T_E_b3f74 : Constant  Value=T_E
  Divide_f15fc : Product  Inputs=*/
  Product_4bea8 : Product
  Product_903f1 : Product
  Blockout_d_E_fd_SG_D_13_44364 : Outport
  wires:
  Constant_-1_49c12/1 -> Product_4bea8/1
  State_E_fd_SG_D_13_5a679/1 -> Product_4bea8/2
  Product_4bea8/1 -> Product_903f1/1
  Constant_K_E_3df9a/1 -> Product_903f1/2
  Constant_T_E_b3f74/1 -> Divide_f15fc/2
  Product_903f1/1 -> Add_3e7a5/1
  State_V_f_SG_D_13_6d482/1 -> Add_3e7a5/2
  Add_3e7a5/1 -> Divide_f15fc/1
  Divide_f15fc/1 -> Blockout_d_E_fd_SG_D_13_44364/1

== system IEEE30_case/SG_D_13/d_Px_1_SG_D_13_block ==
  note: d_Px_1_SG_D_13 in IEEE30_case
      | $\frac{w_{\mathrm{SG},D,13}-2\,\pi \,f_{0}}{T_{w}}-\frac{\mathrm{Px}_{1,\mathrm{SG},D,13}}{T_{w}}$
      | Automatically generated on 2025-11-01 18:35:21 .
  State_Px_1_SG_D_13_cb051 : Inport
  State_w_SG_D_13_74c4a : Inport  Port=2
  Add_0868d : Sum
  Add_fd0a3 : Sum
  Constant_-1_678d1 : Constant  Value=-1
  Constant_-2.0_b50a4 : Constant  Value=-2.0
  Constant_T_w_0ad12 : Constant  Value=T_w
  Constant_T_w_13e33 : Constant  Value=T_w
  Constant_f0_a56c4 : Constant  Value=f0
  Constant_pi_7b263 : Constant  Value=pi
  Divide_09724 : Product  Inputs=*/
  Divide_2b0b4 : Product  Inputs=*/
  Product_32c58 : Product
  Product_33e2f : Product
  Product_a1d4d : Product
  Blockout_d_Px_1_SG_D_13_d2c91 : Outport
  wires:
  Constant_-2.0_b50a4/1 -> Product_a1d4d/1
  Constant_f0_a56c4/1 -> Product_32c58/2
  Constant_pi_7b263/1 -> Product_a1d4d/2
  Product_a1d4d/1 -> Product_32c58/1
  Constant_-1_678d1/1 -> Product_33e2f/1
  Divide_2b0b4/1 -> Add_fd0a3/1
  State_Px_1_SG_D_13_cb051/1 -> Product_33e2f/2
  Constant_T_w_13e33/1 -> Divide_09724/2
  Product_32c58/1 -> Add_0868d/1
  State_w_SG_D_13_74c4a/1 -> Add_0868d/2
  Product_33e2f/1 -> Divide_2b0b4/1
  Constant_T_w_0ad12/1 -> Divide_2b0b4/2
  Add_0868d/1 -> Divide_09724/1
  Divide_09724/1 -> Add_fd0a3/2
  Add_fd0a3/1 -> Blockout_d_Px_1_SG_D_13_d2c91/1

== system IEEE30_case/SG_D_13/d_Px_2_SG_D_13_block ==
  note: d_Px_2_SG_D_13 in IEEE30_case
      | $\frac{\mathrm{Px}_{1,\mathrm{SG},D,13}-T_{2}\,\left(\frac{\mathrm{Px}_{1,\mathrm{SG},D,13}}{T_{w}}-\frac{w_{\mathrm{SG},D,13}-2\,\pi \,f_{0}}{T_{w}}\right)}{T_{1}}-\frac{\mathrm{Px}_{2,\mathrm{SG},D,13}}{T_{1}}$
      | Automatically generated on 2025-11-01 18:35:23 .
  State_Px_2_SG_D_13_19d18 : Inport
  State_Px_1_SG_D_13_fc4bf : Inport  Port=2
  State_Px_1_SG_D_13_6d859 : Inport  Port=3
  State_w_SG_D_13_e5bee : Inport  Port=4
  Add_4dcf5 : Sum
  Add_6ce8b : Sum
  Add_9a5f5 : Sum
  Add_ed697 : Sum
  Constant_-1_a808e : Constant  Value=-1
  Constant_-1_ceccb : Constant  Value=-1
  Constant_-2.0_39bff : Constant  Value=-2.0
  Constant_T_1_70b68 : Constant  Value=T_1
  Constant_T_1_e655d : Constant  Value=T_1
  Constant_T_2_79cd6 : Constant  Value=T_2
  Constant_T_w_2f5ef : Constant  Value=T_w
  Constant_T_w_e95b4 : Constant  Value=T_w
  Constant_f0_4ba57 : Constant  Value=f0
  Constant_pi_263ec : Constant  Value=pi
  Divide_5378a : Product  Inputs=*/
  Divide_6b09c : Product  Inputs=*/
  Divide_8deed : Product  Inputs=*/
  Divide_da5f3 : Product  Inputs=*/
  Product_02a29 : Product
  Product_254dc : Product
  Product_9116b : Product
  Product_c563d : Product
  Product_ee0df : Product
  Blockout_d_Px_2_SG_D_13_f64fc : Outport
  wires:
  Constant_-2.0_39bff/1 -> Product_9116b/1
  Product_9116b/1 -> Product_c563d/1
  Constant_pi_263ec/1 -> Product_9116b/2
  State_Px_1_SG_D_13_fc4bf/1 -> Add_9a5f5/1
  State_Px_1_SG_D_13_6d859/1 -> Product_254dc/2
  Constant_f0_4ba57/1 -> Product_c563d/2
  State_w_SG_D_13_e5bee/1 -> Add_ed697/2
  Product_254dc/1 -> Divide_8deed/1
  Constant_-1_a808e/1 -> Product_254dc/1
  Product_c563d/1 -> Add_ed697/1
  Constant_T_w_2f5ef/1 -> Divide_8deed/2
  Add_ed697/1 -> Divide_6b09c/1
  Constant_T_w_e95b4/1 -> Divide_6b09c/2
  Divide_8deed/1 -> Add_6ce8b/1
  State_Px_2_SG_D_13_19d18/1 -> Product_ee0df/2
  Divide_6b09c/1 -> Add_6ce8b/2
  Constant_T_2_79cd6/1 -> Product_02a29/1
  Add_6ce8b/1 -> Product_02a29/2
  Constant_-1_ceccb/1 -> Product_ee0df/1
  Product_02a29/1 -> Add_9a5f5/2
  Product_ee0df/1 -> Divide_5378a/1
  Constant_T_1_e655d/1 -> Divide_5378a/2
  Add_9a5f5/1 -> Divide_da5f3/1
  Constant_T_1_70b68/1 -> Divide_da5f3/2
  Divide_5378a/1 -> Add_4dcf5/1
  Divide_da5f3/1 -> Add_4dcf5/2
  Add_4dcf5/1 -> Blockout_d_Px_2_SG_D_13_f64fc/1

== system IEEE30_case/SG_D_13/d_Px_3_SG_D_13_block ==
  note: d_Px_3_SG_D_13 in IEEE30_case
      | $\frac{\mathrm{Px}_{2,\mathrm{SG},D,13}+T_{4}\,\left(\frac{\mathrm{Px}_{1,\mathrm{SG},D,13}-T_{2}\,\left(\frac{\mathrm{Px}_{1,\mathrm{SG},D,13}}{T_{w}}-\frac{w_{\mathrm{SG},D,13}-2\,\pi \,f_{0}}{T_{w}}\right)}{T_{1}}-\frac{\mathrm{Px}_{2,\mathrm{SG},D,13}}{T_{1}}\right)}{T_{3}}-\frac{\mathrm{Px}_{3,\mathrm{SG},D,13}}{T_{3}}$
      | Automatically generated on 2025-11-01 18:35:25 .
  State_Px_3_SG_D_13_880e6 : Inport
  State_Px_2_SG_D_13_30d9f : Inport  Port=2
  State_Px_2_SG_D_13_0dea7 : Inport  Port=3
  State_Px_1_SG_D_13_828dc : Inport  Port=4
  State_Px_1_SG_D_13_42a56 : Inport  Port=5
  State_w_SG_D_13_2383e : Inport  Port=6
  Add_30377 : Sum
  Add_4b73f : Sum
  Add_5b22e : Sum
  Add_781bf : Sum
  Add_94d3f : Sum
  Add_d9701 : Sum
  Constant_-1_0e47a : Constant  Value=-1
  Constant_-1_f07f0 : Constant  Value=-1
  Constant_-1_f5737 : Constant  Value=-1
  Constant_-2.0_4ae69 : Constant  Value=-2.0
  Constant_T_1_3e5ec : Constant  Value=T_1
  Constant_T_1_bc889 : Constant  Value=T_1
  Constant_T_2_49f04 : Constant  Value=T_2
  Constant_T_3_15b8b : Constant  Value=T_3
  Constant_T_3_bb4ff : Constant  Value=T_3
  Constant_T_4_043fc : Constant  Value=T_4
  Constant_T_w_41964 : Constant  Value=T_w
  Constant_T_w_c6f73 : Constant  Value=T_w
  Constant_f0_dfa1e : Constant  Value=f0
  Constant_pi_69a99 : Constant  Value=pi
  Divide_01bf9 : Product  Inputs=*/
  Divide_29c48 : Product  Inputs=*/
  Divide_3e8bf : Product  Inputs=*/
  Divide_a0e4b : Product  Inputs=*/
  Divide_c8af2 : Product  Inputs=*/
  Divide_cc926 : Product  Inputs=*/
  Product_0fb3d : Product
  Product_249fc : Product
  Product_886b7 : Product
  Product_9bb29 : Product
  Product_ad57b : Product
  Product_b5b8e : Product
  Product_f2ded : Product
  Blockout_d_Px_3_SG_D_13_010ed : Outport
  wires:
  Constant_-2.0_4ae69/1 -> Product_0fb3d/1
  Product_0fb3d/1 -> Product_f2ded/1
  Constant_pi_69a99/1 -> Product_0fb3d/2
  State_Px_1_SG_D_13_42a56/1 -> Product_249fc/2
  Constant_f0_dfa1e/1 -> Product_f2ded/2
  Product_249fc/1 -> Divide_cc926/1
  Constant_-1_f5737/1 -> Product_249fc/1
  State_w_SG_D_13_2383e/1 -> Add_5b22e/2
  Product_f2ded/1 -> Add_5b22e/1
  Constant_T_w_c6f73/1 -> Divide_cc926/2
  Add_5b22e/1 -> Divide_01bf9/1
  Constant_T_w_41964/1 -> Divide_01bf9/2
  Constant_T_1_3e5ec/1 -> Divide_a0e4b/2
  Divide_cc926/1 -> Add_d9701/1
  Divide_01bf9/1 -> Add_d9701/2
  Constant_T_2_49f04/1 -> Product_9bb29/1
  Add_d9701/1 -> Product_9bb29/2
  Add_781bf/1 -> Blockout_d_Px_3_SG_D_13_010ed/1
  Constant_-1_0e47a/1 -> Product_b5b8e/1
  Divide_c8af2/1 -> Add_781bf/1
  Divide_3e8bf/1 -> Add_94d3f/1
  State_Px_2_SG_D_13_0dea7/1 -> Product_b5b8e/2
  State_Px_1_SG_D_13_828dc/1 -> Add_4b73f/1
  Divide_29c48/1 -> Add_781bf/2
  Constant_T_3_bb4ff/1 -> Divide_c8af2/2
  Product_9bb29/1 -> Add_4b73f/2
  Product_b5b8e/1 -> Divide_3e8bf/1
  Constant_T_4_043fc/1 -> Product_ad57b/1
  Constant_T_1_bc889/1 -> Divide_3e8bf/2
  Add_4b73f/1 -> Divide_a0e4b/1
  Divide_a0e4b/1 -> Add_94d3f/2
  Add_94d3f/1 -> Product_ad57b/2
  Constant_T_3_15b8b/1 -> Divide_29c48/2
  Constant_-1_f07f0/1 -> Product_886b7/1
  State_Px_3_SG_D_13_880e6/1 -> Product_886b7/2
  State_Px_2_SG_D_13_30d9f/1 -> Add_30377/1
  Product_ad57b/1 -> Add_30377/2
  Product_886b7/1 -> Divide_c8af2/1
  Add_30377/1 -> Divide_29c48/1
